simulink model "exercise11NOV"  (R2016a)
settings: Solver=VariableStepAuto  StartTime=0.0  StopTime=10.0  RelTol=1e-3
settings Model: Creator=user  LastModifiedBy=eruffaldi
settings DataIOCC: LimitDataPoints=on
settings DebuggingCC: AllowSymbolicDim=off
settings ModelReferenceCC: PropagateSignalLabelsOutOfModel=off
settings GRTTargetCC: GeneratePreprocessorConditionals=Use local settings

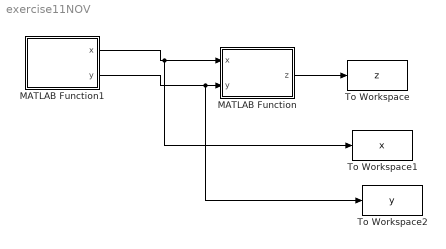
== system exercise11NOV ==
  MATLAB Function : MATLAB Function  TreatAsAtomicUnit=on
  MATLAB Function1 : MATLAB Function  TreatAsAtomicUnit=on
  To Workspace : ToWorkspace  VariableName=z  SaveFormat=Structure With Time  SampleTime=-1
  To Workspace1 : ToWorkspace  VariableName=x  SaveFormat=Structure With Time  SampleTime=-1
  To Workspace2 : ToWorkspace  VariableName=y  SaveFormat=Structure With Time  SampleTime=-1
  wires:
  MATLAB Function/1(z) -> To Workspace/1
  MATLAB Function1/1(x) -> To Workspace1/1, MATLAB Function/1(x)
  MATLAB Function1/2(y) -> To Workspace2/1, MATLAB Function/2(y)

== matlab function exercise11NOV/MATLAB Function1 ==
  data: x output; y output
function [x,y]= esercizio7
%#codegen
[x,y] = meshgrid(-3:0.1:3,-4:0.1:4);
end

== matlab function exercise11NOV/MATLAB Function ==
  data: x input; y input; z output
function z = esercizio7(x,y)
%#codegen
% original spec was: x > 1,  x > 2 & y < 5, otherwise
%
% if we want to keep the semantics we need to go in the reverse order
z = (x+y).^2;
p = x > 2 & y < 5;
z(p) = cos(x(p)).*sin(y(p))+x(p).^2;
p = x > 1;
z(p) = 2*sin(x(p));


end
